simulink model "RL_integralcontrol"  (R2020a)
settings: Solver=VariableStepAuto  StartTime=0.0  StopTime=60  RelTol=1e-3
settings Model: Creator=Ulas  LastModifiedBy=Ulas

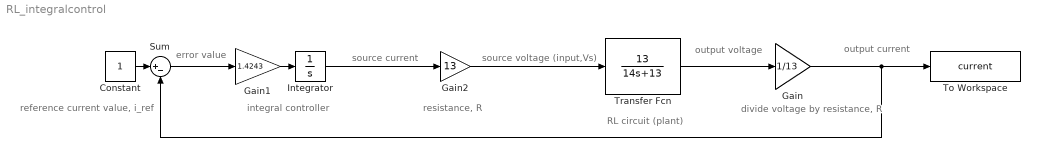
== system RL_integralcontrol ==
  note: output current
  note: output voltage
  note: divide voltage by resistance, R
  note: source voltage (input,Vs)
  note: integral controller
  note: RL circuit (plant)
  note: error value
  note: reference current value, i_ref
  note: resistance, R
  note: source current
  Constant : Constant
  Gain : Gain  Gain=1/13
  Gain1 : Gain  Gain=1.4243
  Gain2 : Gain  Gain=13
  Integrator : Integrator
  Sum : Sum  Inputs=|+-
  To Workspace : ToWorkspace  VariableName=current  SaveFormat=Timeseries  SampleTime=-1
  Transfer Fcn : TransferFcn  Numerator=[13]  Denominator=[14 13]
  wires:
  Constant/1 -> Sum/1
  Integrator/1 -> Gain2/1
  Transfer Fcn/1 -> Gain/1
  Gain/1 -> To Workspace/1, Sum/2
  Sum/1 -> Gain1/1
  Gain1/1 -> Integrator/1
  Gain2/1 -> Transfer Fcn/1
